simulink model "firmware"  (R2020a)
settings: Solver=FixedStepAuto  StartTime=0.0  StopTime=10.0  FixedStep=1e-3  RelTol=1e-3  EnableMultiTasking=on
undefined symbols (not defined in the file): A0, A1, D0, D1, D10, D11, D12, D13, D2, D3, D4, D5, D6, D7, D8, D9, magnitude, PTA0, PTA1, PTA2, PTB2, PTB23, PTB3, PTB9, PTC16, PTC17, PTC2, PTC3, PTC4, PTD0, PTD1, PTD2, PTD3
libraries: etargetslib x35, frdmk64flib x23, dspstat3 x1
(part 1 of 2)
settings Model: ExtModeTrigDuration=5  Creator=eotte  LastModifiedBy=rafit
settings OptimizationCC: EnhancedBackFolding=on  PassReuseOutputArgsAs=Individual arguments  ZeroExternalMemoryAtStartup=off  ZeroInternalMemoryAtStartup=off  MaxStackSize=64  OptimizeBlockOrder=speed  DifferentSizesBufferReuse=on  OptimizationCustomize=off  EfficientTunableParamExpr=on
settings DebuggingCC: ParameterTunabilityLossMsg=error
settings HardwareCC: ProdBitPerPointer=32  ProdBitPerSizeT=32  ProdBitPerPtrDiffT=32  ProdLargestAtomicInteger=Long  ProdLargestAtomicFloat=Double  ProdWordSize=32  ProdHWDeviceType=ARM Compatible->ARM Cortex
settings SFSimCC: MATLABDynamicMemAlloc=off
settings RTWCC: SystemTargetFile=ert.tlc  HardwareBoard=NXP FRDM-K64F  TemplateMakefile=ert_default_tmf  Toolchain=GNU Tools for ARM Embedded Processors
settings CodeAppCC: ForceParamTrailComments=on  IgnoreCustomStorageClasses=off  OperatorAnnotations=on  SimulinkDataObjDesc=on  SFDataObjDesc=on  InsertBlockDesc=on

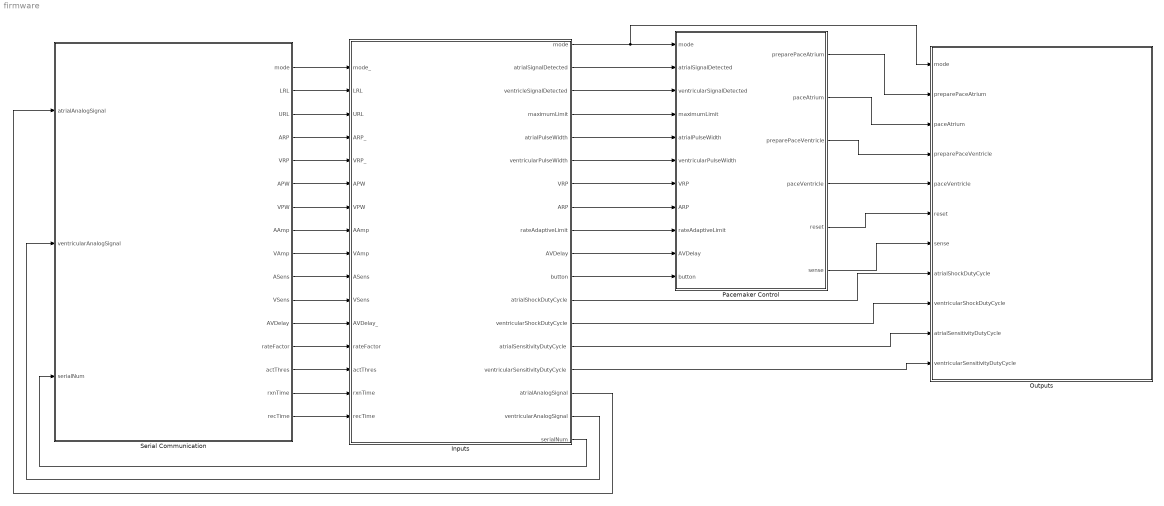
== system firmware ==
  Inputs : Subsystem
  Outputs : Subsystem
  Pacemaker Control : Stateflow chart  TreatAsAtomicUnit=on
  Serial Communication : Subsystem
  wires:
  Pacemaker Control/1(preparePaceAtrium) -> Outputs/2(preparePaceAtrium)
  Pacemaker Control/3(preparePaceVentricle) -> Outputs/4(preparePaceVentricle)
  Pacemaker Control/2(paceAtrium) -> Outputs/3(paceAtrium)
  Pacemaker Control/4(paceVentricle) -> Outputs/5(paceVentricle)
  Inputs/1(mode) -> Pacemaker Control/1(mode), Outputs/1(mode)
  Pacemaker Control/5(reset) -> Outputs/6(reset)
  Inputs/2(atrialSignalDetected) -> Pacemaker Control/2(atrialSignalDetected)
  Inputs/3(ventricleSignalDetected) -> Pacemaker Control/3(ventricularSignalDetected)
  Inputs/15(ventricularSensitivityDutyCycle) -> Outputs/11(ventricularSensitivityDutyCycle)
  Inputs/14(atrialSensitivityDutyCycle) -> Outputs/10(atrialSensitivityDutyCycle)
  Inputs/13(ventricularShockDutyCycle) -> Outputs/9(ventricularShockDutyCycle)
  Inputs/12(atrialShockDutyCycle) -> Outputs/8(atrialShockDutyCycle)
  Inputs/4(maximumLimit) -> Pacemaker Control/4(maximumLimit)
  Inputs/5(atrialPulseWidth) -> Pacemaker Control/5(atrialPulseWidth)
  Inputs/6(ventricularPulseWidth) -> Pacemaker Control/6(ventricularPulseWidth)
  Inputs/7(VRP) -> Pacemaker Control/7(VRP)
  Inputs/8(ARP) -> Pacemaker Control/8(ARP)
  Pacemaker Control/6(sense) -> Outputs/7(sense)
  Serial Communication/1(mode) -> Inputs/1(mode_)
  Serial Communication/2(LRL) -> Inputs/2(LRL)
  Serial Communication/3(URL) -> Inputs/3(URL)
  Serial Communication/4(ARP) -> Inputs/4(ARP_)
  Serial Communication/5(VRP) -> Inputs/5(VRP_)
  Serial Communication/6(APW) -> Inputs/6(APW)
  Serial Communication/7(VPW) -> Inputs/7(VPW)
  Serial Communication/8(AAmp) -> Inputs/8(AAmp)
  Serial Communication/9(VAmp) -> Inputs/9(VAmp)
  Serial Communication/10(ASens) -> Inputs/10(ASens)
  Serial Communication/11(VSens) -> Inputs/11(VSens)
  Inputs/18(serialNum) -> Serial Communication/3(serialNum)
  Inputs/17(ventricularAnalogSignal) -> Serial Communication/2(ventricularAnalogSignal)
  Inputs/16(atrialAnalogSignal) -> Serial Communication/1(atrialAnalogSignal)
  Serial Communication/12(AVDelay) -> Inputs/12(AVDelay_)
  Serial Communication/13(rateFactor) -> Inputs/13(rateFactor)
  Serial Communication/14(actThres) -> Inputs/14(actThres)
  Serial Communication/15(rxnTime) -> Inputs/15(rxnTime)
  Serial Communication/16(recTime) -> Inputs/16(recTime)
  Inputs/9(rateAdaptiveLimit) -> Pacemaker Control/9(rateAdaptiveLimit)
  Inputs/10(AVDelay) -> Pacemaker Control/10(AVDelay)
  Inputs/11(button) -> Pacemaker Control/11(button)

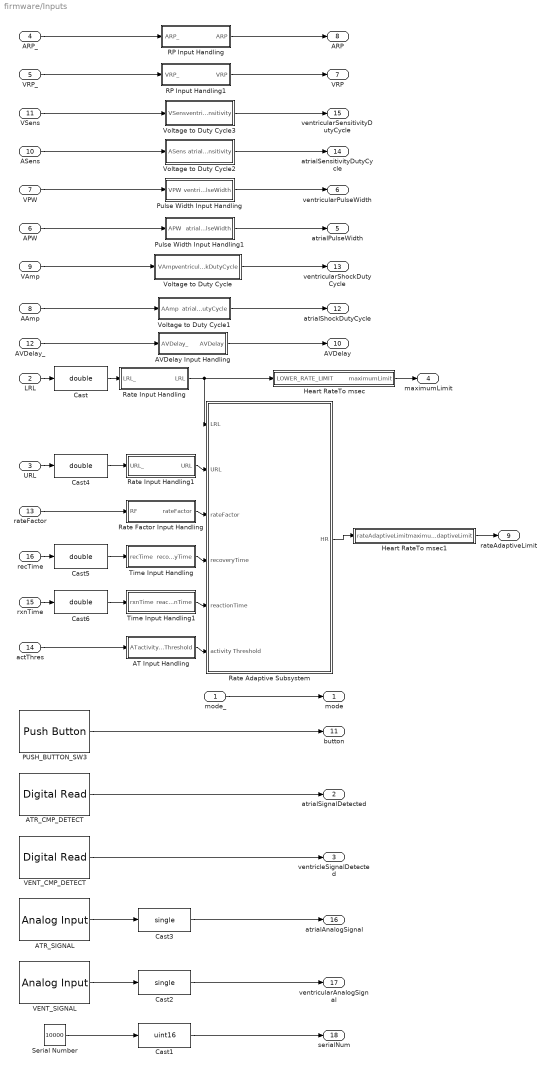
== system firmware/Inputs ==
  mode_ : Inport
  LRL : Inport  Port=2
  URL : Inport  Port=3
  ARP_ : Inport  Port=4
  VRP_ : Inport  Port=5
  APW : Inport  Port=6
  VPW : Inport  Port=7
  AAmp : Inport  Port=8
  VAmp : Inport  Port=9
  ASens : Inport  Port=10
  VSens : Inport  Port=11
  AVDelay_ : Inport  Port=12
  rateFactor : Inport  Port=13
  actThres : Inport  Port=14
  rxnTime : Inport  Port=15
  recTime : Inport  Port=16
  AT Input Handling : Subsystem
  ATR_CMP_DETECT : frdmk64flib/Digital Read  Whichpin=PTC16 (D0)  SampleTime=-1
  ATR_SIGNAL : frdmk64flib/Analog Input  Whichpin=PTB2 (A0)  SampleTime=-1
  AVDelay Input Handling : Subsystem
  Cast{,4..6} (4 alike) : DataTypeConversion  OutDataTypeStr=double  RndMeth=Nearest
  Cast1 : DataTypeConversion  OutDataTypeStr=uint16  RndMeth=Nearest
  Cast2 : DataTypeConversion  OutDataTypeStr=single  RndMeth=Nearest
  Cast3 : DataTypeConversion  OutDataTypeStr=single  RndMeth=Nearest
  Heart RateTo msec : Subsystem
  Heart RateTo msec1 : Subsystem
  PUSH_BUTTON_SW3 : frdmk64flib/Push Button  Whichswitch=SW3  SampleTime1=-1
  Pulse Width Input Handling : Subsystem
  Pulse Width Input Handling1 : Subsystem
  RP Input Handling : Subsystem
  RP Input Handling1 : Subsystem
  Rate Adaptive Subsystem : Subsystem
  Rate Factor Input Handling : Subsystem
  Rate Input Handling : Subsystem
  Rate Input Handling1 : Subsystem
  Serial Number : Constant  Value=10000
  Time Input Handling : Subsystem
  Time Input Handling1 : Subsystem
  VENT_CMP_DETECT : frdmk64flib/Digital Read  Whichpin=PTC17 (D1)  SampleTime=-1
  VENT_SIGNAL : frdmk64flib/Analog Input  Whichpin=PTB3 (A1)  SampleTime=-1
  Voltage to Duty Cycle : Subsystem
  Voltage to Duty Cycle1 : Subsystem
  Voltage to Duty Cycle2 : Subsystem
  Voltage to Duty Cycle3 : Subsystem
  mode : Outport
  atrialSignalDetected : Outport  Port=2
  ventricleSignalDetected : Outport  Port=3
  maximumLimit : Outport  Port=4
  atrialPulseWidth : Outport  Port=5
  ventricularPulseWidth : Outport  Port=6
  VRP : Outport  Port=7
  ARP : Outport  Port=8
  rateAdaptiveLimit : Outport  Port=9
  AVDelay : Outport  Port=10
  button : Outport  Port=11
  atrialShockDutyCycle : Outport  Port=12
  ventricularShockDutyCycle : Outport  Port=13
  atrialSensitivityDutyCycle : Outport  Port=14
  ventricularSensitivityDutyCycle : Outport  Port=15
  atrialAnalogSignal : Outport  Port=16
  ventricularAnalogSignal : Outport  Port=17
  serialNum : Outport  Port=18
  wires:
  mode_/1 -> mode/1
  ATR_CMP_DETECT/1 -> atrialSignalDetected/1
  VENT_CMP_DETECT/1 -> ventricleSignalDetected/1
  AAmp/1 -> Voltage to Duty Cycle1/1(AAmp)
  VAmp/1 -> Voltage to Duty Cycle/1(VAmp)
  VSens/1 -> Voltage to Duty Cycle3/1(VSens)
  ASens/1 -> Voltage to Duty Cycle2/1(ASens)
  VPW/1 -> Pulse Width Input Handling/1(VPW)
  Heart RateTo msec/1(maximumLimit) -> maximumLimit/1
  Voltage to Duty Cycle/1(ventricularShockDutyCycle) -> ventricularShockDutyCycle/1
  Voltage to Duty Cycle1/1(atrialShockDutyCycle) -> atrialShockDutyCycle/1
  Voltage to Duty Cycle3/1(ventricularSensitivity) -> ventricularSensitivityDutyCycle/1
  Voltage to Duty Cycle2/1(atrialSensitivity) -> atrialSensitivityDutyCycle/1
  Pulse Width Input Handling/1(ventricularPulseWidth) -> ventricularPulseWidth/1
  Pulse Width Input Handling1/1(atrialPulseWidth) -> atrialPulseWidth/1
  APW/1 -> Pulse Width Input Handling1/1(APW)
  RP Input Handling1/1(VRP) -> VRP/1
  RP Input Handling/1(ARP) -> ARP/1
  ARP_/1 -> RP Input Handling/1(ARP_)
  VRP_/1 -> RP Input Handling1/1(VRP_)
  Serial Number/1 -> Cast1/1
  ATR_SIGNAL/1 -> Cast3/1
  VENT_SIGNAL/1 -> Cast2/1
  Cast1/1 -> serialNum/1
  Cast2/1 -> ventricularAnalogSignal/1
  Cast3/1 -> atrialAnalogSignal/1
  rateFactor/1 -> Rate Factor Input Handling/1(RF)
  actThres/1 -> AT Input Handling/1(AT)
  Rate Adaptive Subsystem/1(HR) -> Heart RateTo msec1/1(rateAdaptiveLimit)
  Heart RateTo msec1/1(maximumAdaptiveLimit) -> rateAdaptiveLimit/1
  AVDelay_/1 -> AVDelay Input Handling/1(AVDelay_)
  PUSH_BUTTON_SW3/1 -> button/1
  AVDelay Input Handling/1(AVDelay) -> AVDelay/1
  LRL/1 -> Cast/1
  Cast/1 -> Rate Input Handling/1(LRL_)
  Rate Input Handling/1(LRL) -> Heart RateTo msec/1(LOWER_RATE_LIMIT), Rate Adaptive Subsystem/1(LRL)
  Cast4/1 -> Rate Input Handling1/1(URL_)
  Rate Input Handling1/1(URL) -> Rate Adaptive Subsystem/2(URL)
  URL/1 -> Cast4/1
  Rate Factor Input Handling/1(rateFactor) -> Rate Adaptive Subsystem/3(rateFactor)
  Time Input Handling/1(recoveryTime) -> Rate Adaptive Subsystem/4(recoveryTime)
  Time Input Handling1/1(reactionTime) -> Rate Adaptive Subsystem/5(reactionTime)
  AT Input Handling/1(activityThreshold) -> Rate Adaptive Subsystem/6(activity Threshold)
  Cast5/1 -> Time Input Handling/1(recTime)
  recTime/1 -> Cast5/1
  Cast6/1 -> Time Input Handling1/1(rxnTime)
  rxnTime/1 -> Cast6/1

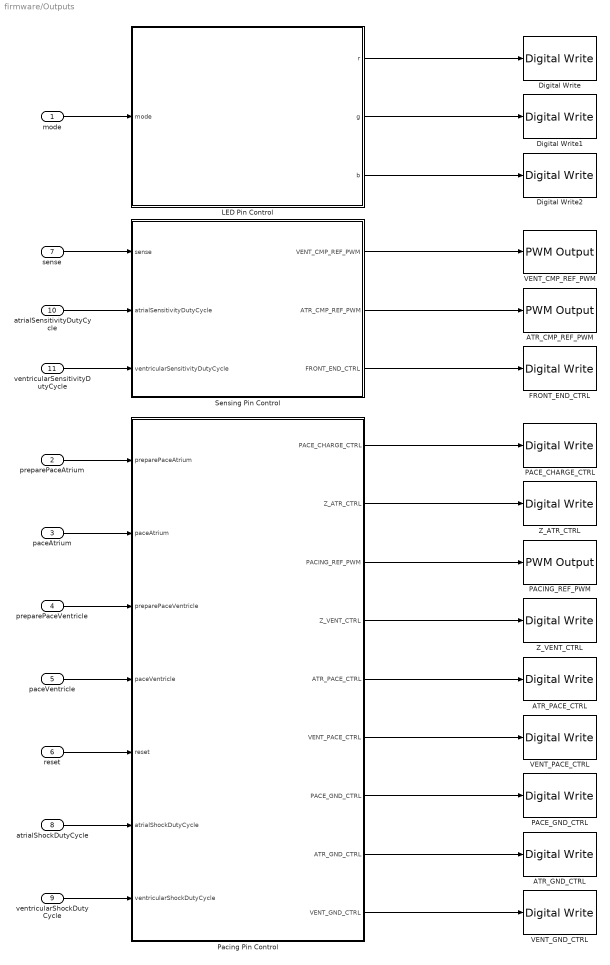
== system firmware/Outputs ==
  mode : Inport
  preparePaceAtrium : Inport  Port=2
  paceAtrium : Inport  Port=3
  preparePaceVentricle : Inport  Port=4
  paceVentricle : Inport  Port=5
  reset : Inport  Port=6
  sense : Inport  Port=7
  atrialShockDutyCycle : Inport  Port=8
  ventricularShockDutyCycle : Inport  Port=9
  atrialSensitivityDutyCycle : Inport  Port=10
  ventricularSensitivityDutyCycle : Inport  Port=11
  ATR_CMP_REF_PWM : frdmk64flib/PWM Output  Whichpin=PTC2 (D6)  InitialFrequency=2000  InitialDutyCycle=0
  ATR_GND_CTRL : frdmk64flib/Digital Write  Whichpin=PTD2 (D11)
  ATR_PACE_CTRL : frdmk64flib/Digital Write  Whichpin=PTA0 (D8)
  Digital Write : frdmk64flib/Digital Write  Whichpin=RED_LED
  Digital Write1 : frdmk64flib/Digital Write  Whichpin=GREEN_LED
  Digital Write2 : frdmk64flib/Digital Write  Whichpin=BLUE_LED
  FRONT_END_CTRL : frdmk64flib/Digital Write  Whichpin=PTD1 (D13)
  LED Pin Control : Stateflow chart  TreatAsAtomicUnit=on
  PACE_CHARGE_CTRL : frdmk64flib/Digital Write  Whichpin=PTB9 (D2)
  PACE_GND_CTRL : frdmk64flib/Digital Write  Whichpin=PTD0 (D10)
  PACING_REF_PWM : frdmk64flib/PWM Output  Whichpin=PTA2 (D5)  InitialFrequency=2000  InitialDutyCycle=0
  Pacing Pin Control : Stateflow chart  TreatAsAtomicUnit=on
      settings: PortSchema="{\"entries\":[{\"content\":{\"sides\":[{\"content\":{\"connectorIds\":[\"In1\",\"In2\",\"In3\",\"In4\",\"In5\",\"In6\",\"In7\"]},\"type\":\"ConnectorPlacement.EquallySpacedRectSide\",\"uuid\":\"92253962-87e9-4e7c-bcdb-24e58fe0c055\"},{\"content\":{\"connectorIds\":[\"Out2\",\"Out8\",\"Out5\",\"Out9\",\"Out3\",\"Out7\",\"Out4\",\"Out1\",\"Out6\"],\"side\":\"RIGHT\"},\"type\":\"ConnectorPlacement.EquallySpacedRectSide\",\"uuid\":\"4cb9541d-32ff-4bb4-8e4b-d9f1d7e76c76\"},{\"content\":{\"connectorIds\":[],\"side\":\"TOP\"},\"type\":\"ConnectorPlacement.EquallySpacedRectSide\",\"uuid\":\"cc690cb9-25b8-4ee8-ae3f-a22909f5e3a8\"},{\"content\":{\"connectorIds\":[],\"side\":\"BOTTOM\"},\"type\":\"ConnectorPlacement.EquallySpacedRectSide\",\"uuid\":\"0aa6c860-c953-4b2e-baf5-040a508b9d07\"}]},\"type\":\"ConnectorPlacement.EquallySpacedConnector\",\"uuid\":\"d7c6b2d5-ade3-439b-b1ea-d68e76d328ac\"}],\"packageUris\":[\"http://schema.mathworks.com/mf0/Connector/19700101\"],\"version\":\"1.0\"}"
  Sensing Pin Control : Stateflow chart  TreatAsAtomicUnit=on
      settings: PortSchema="{\"entries\":[{\"content\":{\"sides\":[{\"content\":{\"connectorIds\":[\"In1\",\"In2\",\"In3\"]},\"type\":\"ConnectorPlacement.EquallySpacedRectSide\",\"uuid\":\"f0f6a072-4109-4fa4-bc82-6d6350130513\"},{\"content\":{\"connectorIds\":[\"Out3\",\"Out2\",\"Out1\"],\"side\":\"RIGHT\"},\"type\":\"ConnectorPlacement.EquallySpacedRectSide\",\"uuid\":\"04a191da-9ef7-404f-bbc7-e2275fa0f798\"},{\"content\":{\"connectorIds\":[],\"side\":\"TOP\"},\"type\":\"ConnectorPlacement.EquallySpacedRectSide\",\"uuid\":\"3258143e-ec04-4818-a8fd-7397dd93120a\"}]},\"type\":\"ConnectorPlacement.EquallySpacedConnector\",\"uuid\":\"abd9187b-7230-471c-b20b-6fa4748c984d\"}],\"packageUris\":[\"http://schema.mathworks.com/mf0/Connector/19700101\"],\"version\":\"1.0\"}"
  VENT_CMP_REF_PWM : frdmk64flib/PWM Output  Whichpin=PTA1 (D3)  InitialFrequency=2000  InitialDutyCycle=0
  VENT_GND_CTRL : frdmk64flib/Digital Write  Whichpin=PTD3 (D12)
  VENT_PACE_CTRL : frdmk64flib/Digital Write  Whichpin=PTC4 (D9)
  Z_ATR_CTRL : frdmk64flib/Digital Write  Whichpin=PTB23 (D4)
  Z_VENT_CTRL : frdmk64flib/Digital Write  Whichpin=PTC3 (D7)
  wires:
  preparePaceAtrium/1 -> Pacing Pin Control/1(preparePaceAtrium)
  paceAtrium/1 -> Pacing Pin Control/2(paceAtrium)
  preparePaceVentricle/1 -> Pacing Pin Control/3(preparePaceVentricle)
  paceVentricle/1 -> Pacing Pin Control/4(paceVentricle)
  Pacing Pin Control/1(ATR_GND_CTRL) -> ATR_GND_CTRL/1
  Pacing Pin Control/2(PACE_CHARGE_CTRL) -> PACE_CHARGE_CTRL/1
  Pacing Pin Control/3(ATR_PACE_CTRL) -> ATR_PACE_CTRL/1
  Pacing Pin Control/5(PACING_REF_PWM) -> PACING_REF_PWM/1
  Pacing Pin Control/8(Z_ATR_CTRL) -> Z_ATR_CTRL/1
  Pacing Pin Control/4(PACE_GND_CTRL) -> PACE_GND_CTRL/1
  Pacing Pin Control/6(VENT_GND_CTRL) -> VENT_GND_CTRL/1
  Pacing Pin Control/9(Z_VENT_CTRL) -> Z_VENT_CTRL/1
  Pacing Pin Control/7(VENT_PACE_CTRL) -> VENT_PACE_CTRL/1
  reset/1 -> Pacing Pin Control/5(reset)
  atrialShockDutyCycle/1 -> Pacing Pin Control/6(atrialShockDutyCycle)
  ventricularShockDutyCycle/1 -> Pacing Pin Control/7(ventricularShockDutyCycle)
  LED Pin Control/2(g) -> Digital Write1/1
  LED Pin Control/1(r) -> Digital Write/1
  LED Pin Control/3(b) -> Digital Write2/1
  mode/1 -> LED Pin Control/1(mode)
  sense/1 -> Sensing Pin Control/1(sense)
  atrialSensitivityDutyCycle/1 -> Sensing Pin Control/2(atrialSensitivityDutyCycle)
  ventricularSensitivityDutyCycle/1 -> Sensing Pin Control/3(ventricularSensitivityDutyCycle)
  Sensing Pin Control/1(FRONT_END_CTRL) -> FRONT_END_CTRL/1
  Sensing Pin Control/2(ATR_CMP_REF_PWM) -> ATR_CMP_REF_PWM/1
  Sensing Pin Control/3(VENT_CMP_REF_PWM) -> VENT_CMP_REF_PWM/1

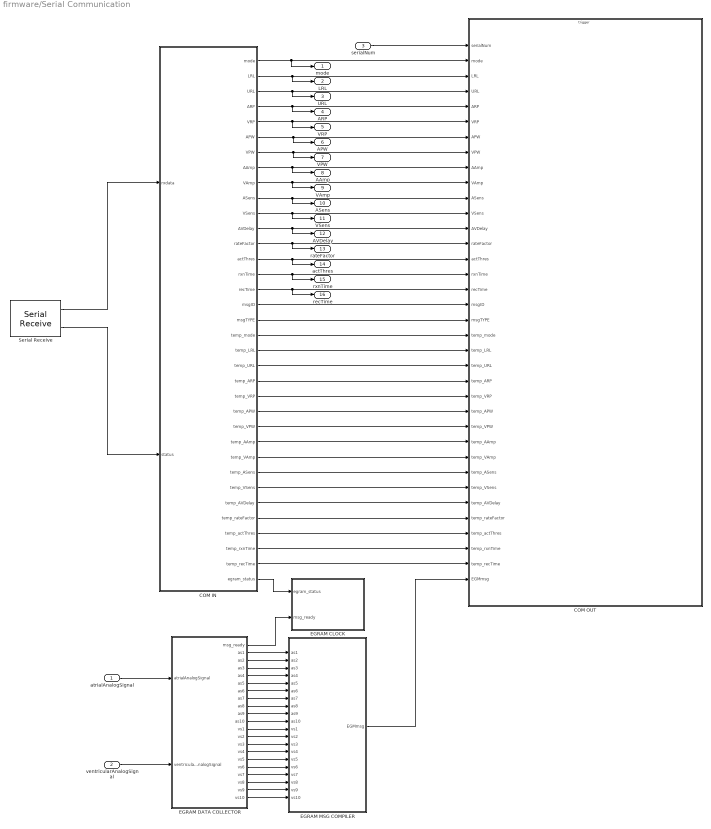
== system firmware/Serial Communication ==
  atrialAnalogSignal : Inport
  ventricularAnalogSignal : Inport  Port=2
  serialNum : Inport  Port=3
  COM IN : Stateflow chart  TreatAsAtomicUnit=on
      settings: PortSchema="{\"entries\":[{\"content\":{\"sides\":[{\"content\":{\"connectorIds\":[\"In1\",\"In2\"]},\"type\":\"ConnectorPlacement.EquallySpacedRectSide\",\"uuid\":\"2e8e9e18-d37c-4b73-b0dd-3e22f2864207\"},{\"content\":{\"connectorIds\":[\"Out1\",\"Out2\",\"Out3\",\"Out4\",\"Out5\",\"Out6\",\"Out7\",\"Out8\",\"Out9\",\"Out10\",\"Out11\",\"Out12\",\"Out13\",\"Out14\",\"Out15\",\"Out16\",\"Out28\",\"Out29\",\"Out17\",\"Out18\",\"Out19\",\"Out20\",\"Out21\",\"Out22\",\"Out23\",\"Out24\",\"Out25\",\"Out26\",\"Out27\",\"Out30\",\"Out31\",\"Out32\",\"Out33\",\"Out34\",\"Out35\"],\"side\":\"RIGHT\"},\"type\":\"ConnectorPlacement.EquallySpacedRectSide\",\"uuid\":\"4c9bee01-a377-43c4-9bd2-1da39583f7b1\"},{\"content\":{\"connectorIds\":[],\"side\":\"TOP\"},\"type\":\"ConnectorPlacement.EquallySpacedRectSide\",\"uuid\":\"f3e8c630-a6ea-4f37-b829-1068b53873bf\"},{\"content\":{\"connectorIds\":[],\"side\":\"BOTTOM\"},\"type\":\"ConnectorPlacement.EquallySpacedRectSide\",\"uuid\":\"e2f98f06-b9c7-4ad9-9fdf-47a7e91a95c4\"}]},\"type\":\"ConnectorPlacement.EquallySpacedConnector\",\"uuid\":\"8e1bc096-629b-4ab2-88c2-6836d8378271\"}],\"packageUris\":[\"http://schema.mathworks.com/mf0/Connector/19700101\"],\"version\":\"1.0\"}"
  COM OUT : Subsystem  TreatAsAtomicUnit=on
  EGRAM CLOCK : Stateflow chart  TreatAsAtomicUnit=on
  EGRAM DATA COLLECTOR : Stateflow chart  TreatAsAtomicUnit=on
      settings: PortSchema="{\"entries\":[{\"content\":{\"sides\":[{\"content\":{\"connectorIds\":[\"In1\",\"In2\"]},\"type\":\"ConnectorPlacement.EquallySpacedRectSide\",\"uuid\":\"97e1670e-7108-4d44-b2cd-721317f0ea01\"},{\"content\":{\"connectorIds\":[\"Out1\",\"Out2\",\"Out3\",\"Out4\",\"Out9\",\"Out10\",\"Out11\",\"Out12\",\"Out13\",\"Out14\",\"Out8\",\"Out5\",\"Out6\",\"Out7\",\"Out16\",\"Out17\",\"Out18\",\"Out19\",\"Out20\",\"Out21\",\"Out15\"],\"side\":\"RIGHT\"},\"type\":\"ConnectorPlacement.EquallySpacedRectSide\",\"uuid\":\"43d6a441-c68e-4a27-91a0-990e1296c4d1\"},{\"content\":{\"connectorIds\":[],\"side\":\"TOP\"},\"type\":\"ConnectorPlacement.EquallySpacedRectSide\",\"uuid\":\"c7be9cee-947c-49b5-a7f8-da78c79fbdaa\"}]},\"type\":\"ConnectorPlacement.EquallySpacedConnector\",\"uuid\":\"a175dd55-c9cb-4f10-b1e9-b74267d4f2a4\"}],\"packageUris\":[\"http://schema.mathworks.com/mf0/Connector/19700101\"],\"version\":\"1.0\"}"
  EGRAM MSG COMPILER : Subsystem
  Serial Receive : frdmk64flib/Serial Receive  SCIModule=0  Baudrate=uint32(9600)  Parity=None  StopBits=1  HardwareFlowControl=None  ByteOrder=LittleEndian  DataType=uint8  DataLength=82  BlockingMode=off  OutputStatus=on  SampleTime=-1
  mode : Outport
  LRL : Outport  Port=2
  URL : Outport  Port=3
  ARP : Outport  Port=4
  VRP : Outport  Port=5
  APW : Outport  Port=6
  VPW : Outport  Port=7
  AAmp : Outport  Port=8
  VAmp : Outport  Port=9
  ASens : Outport  Port=10
  VSens : Outport  Port=11
  AVDelay : Outport  Port=12
  rateFactor : Outport  Port=13
  actThres : Outport  Port=14
  rxnTime : Outport  Port=15
  recTime : Outport  Port=16
  wires:
  Serial Receive/1 -> COM IN/1(rxdata)
  Serial Receive/2 -> COM IN/2(status)
  COM IN/17(temp_mode) -> COM OUT/20(temp_mode)
  COM IN/18(temp_LRL) -> COM OUT/21(temp_LRL)
  COM IN/7(VPW) -> VPW/1, COM OUT/8(VPW)
  COM IN/28(msgID) -> COM OUT/18(msgID)
  COM IN/29(msgTYPE) -> COM OUT/19(msgTYPE)
  COM IN/19(temp_URL) -> COM OUT/22(temp_URL)
  COM IN/20(temp_ARP) -> COM OUT/23(temp_ARP)
  COM IN/21(temp_VRP) -> COM OUT/24(temp_VRP)
  COM IN/22(temp_APW) -> COM OUT/25(temp_APW)
  COM IN/23(temp_VPW) -> COM OUT/26(temp_VPW)
  COM IN/24(temp_AAmp) -> COM OUT/27(temp_AAmp)
  COM IN/25(temp_VAmp) -> COM OUT/28(temp_VAmp)
  COM IN/26(temp_ASens) -> COM OUT/29(temp_ASens)
  COM IN/27(temp_VSens) -> COM OUT/30(temp_VSens)
  serialNum/1 -> COM OUT/1(serialNum)
  atrialAnalogSignal/1 -> EGRAM DATA COLLECTOR/1(atrialAnalogSignal)
  ventricularAnalogSignal/1 -> EGRAM DATA COLLECTOR/2(ventricularAnalogSignal)
  EGRAM DATA COLLECTOR/1(msg_ready) -> EGRAM CLOCK/2(msg_ready)
  EGRAM MSG COMPILER/1(EGMmsg) -> COM OUT/36(EGMmsg)
  EGRAM DATA COLLECTOR/2(as1) -> EGRAM MSG COMPILER/1(as1)
  EGRAM DATA COLLECTOR/3(as2) -> EGRAM MSG COMPILER/2(as2)
  EGRAM DATA COLLECTOR/4(as3) -> EGRAM MSG COMPILER/3(as3)
  EGRAM DATA COLLECTOR/5(vs1) -> EGRAM MSG COMPILER/11(vs1)
  EGRAM DATA COLLECTOR/6(vs2) -> EGRAM MSG COMPILER/12(vs2)
  EGRAM DATA COLLECTOR/7(vs3) -> EGRAM MSG COMPILER/13(vs3)
  COM IN/35(egram_status) -> EGRAM CLOCK/1(egram_status)
  EGRAM DATA COLLECTOR/9(as4) -> EGRAM MSG COMPILER/4(as4)
  EGRAM DATA COLLECTOR/10(as5) -> EGRAM MSG COMPILER/5(as5)
  EGRAM DATA COLLECTOR/11(as6) -> EGRAM MSG COMPILER/6(as6)
  EGRAM DATA COLLECTOR/12(as7) -> EGRAM MSG COMPILER/7(as7)
  EGRAM DATA COLLECTOR/13(as8) -> EGRAM MSG COMPILER/8(as8)
  EGRAM DATA COLLECTOR/14(as9) -> EGRAM MSG COMPILER/9(as9)
  EGRAM DATA COLLECTOR/8(as10) -> EGRAM MSG COMPILER/10(as10)
  EGRAM DATA COLLECTOR/16(vs4) -> EGRAM MSG COMPILER/14(vs4)
  EGRAM DATA COLLECTOR/17(vs5) -> EGRAM MSG COMPILER/15(vs5)
  EGRAM DATA COLLECTOR/18(vs6) -> EGRAM MSG COMPILER/16(vs6)
  EGRAM DATA COLLECTOR/19(vs7) -> EGRAM MSG COMPILER/17(vs7)
  EGRAM DATA COLLECTOR/20(vs8) -> EGRAM MSG COMPILER/18(vs8)
  EGRAM DATA COLLECTOR/21(vs9) -> EGRAM MSG COMPILER/19(vs9)
  EGRAM DATA COLLECTOR/15(vs10) -> EGRAM MSG COMPILER/20(vs10)
  COM IN/1(mode) -> mode/1, COM OUT/2(mode)
  COM IN/2(LRL) -> LRL/1, COM OUT/3(LRL)
  COM IN/3(URL) -> URL/1, COM OUT/4(URL)
  COM IN/4(ARP) -> ARP/1, COM OUT/5(ARP)
  COM IN/5(VRP) -> VRP/1, COM OUT/6(VRP)
  COM IN/6(APW) -> APW/1, COM OUT/7(APW)
  COM IN/8(AAmp) -> AAmp/1, COM OUT/9(AAmp)
  COM IN/9(VAmp) -> VAmp/1, COM OUT/10(VAmp)
  COM IN/10(ASens) -> COM OUT/11(ASens), ASens/1
  COM IN/11(VSens) -> VSens/1, COM OUT/12(VSens)
  COM IN/12(AVDelay) -> AVDelay/1, COM OUT/13(AVDelay)
  COM IN/13(rateFactor) -> rateFactor/1, COM OUT/14(rateFactor)
  COM IN/14(actThres) -> actThres/1, COM OUT/15(actThres)
  COM IN/15(rxnTime) -> rxnTime/1, COM OUT/16(rxnTime)
  COM IN/16(recTime) -> recTime/1, COM OUT/17(recTime)
  COM IN/30(temp_AVDelay) -> COM OUT/31(temp_AVDelay)
  COM IN/31(temp_rateFactor) -> COM OUT/32(temp_rateFactor)
  COM IN/32(temp_actThres) -> COM OUT/33(temp_actThres)
  COM IN/33(temp_rxnTime) -> COM OUT/34(temp_rxnTime)
  COM IN/34(temp_recTime) -> COM OUT/35(temp_recTime)

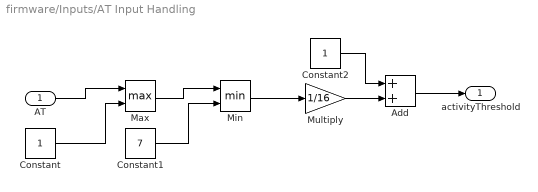
== system firmware/Inputs/AT Input Handling ==
  AT : Inport
  Add : Sum
  Constant : Constant
  Constant1 : Constant  Value=7
  Constant2 : Constant
  Max : MinMax  Function=max  Inputs=2
  Min : MinMax  Inputs=2
  Multiply : Gain  Gain=1/16
  activityThreshold : Outport
  wires:
  Max/1 -> Min/1
  AT/1 -> Max/1
  Min/1 -> Multiply/1
  Constant/1 -> Max/2
  Constant1/1 -> Min/2
  Constant2/1 -> Add/1
  Multiply/1 -> Add/2
  Add/1 -> activityThreshold/1

== system firmware/Inputs/AVDelay Input Handling ==
  AVDelay_ : Inport
  Constant : Constant  Value=30
  Constant1 : Constant  Value=300
  Max : MinMax  Function=max  Inputs=2
  Min : MinMax  Inputs=2
  AVDelay : Outport
  wires:
  Max/1 -> Min/1
  AVDelay_/1 -> Max/1
  Min/1 -> AVDelay/1
  Constant/1 -> Max/2
  Constant1/1 -> Min/2

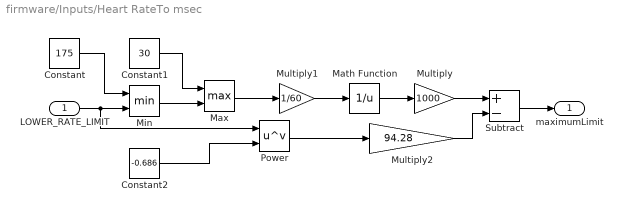
== system firmware/Inputs/Heart RateTo msec ==
  LOWER_RATE_LIMIT : Inport
  Constant : Constant  Value=175
  Constant1 : Constant  Value=30
  Constant2 : Constant  Value=-0.686
  Math Function : Math  Operator=reciprocal  SaturateOnIntegerOverflow=on
  Max : MinMax  Function=max  Inputs=2
  Min : MinMax  Inputs=2
  Multiply : Gain  Gain=1000
  Multiply1 : Gain  Gain=1/60
  Multiply2 : Gain  Gain=94.28
  Power : Math  Operator=pow  OutputSignalType=real  SaturateOnIntegerOverflow=on
  Subtract : Sum  Inputs=+-
  maximumLimit : Outport
  wires:
  Multiply1/1 -> Math Function/1
  Multiply/1 -> Subtract/1
  LOWER_RATE_LIMIT/1 -> Power/1, Min/2
  Min/1 -> Max/2
  Max/1 -> Multiply1/1
  Constant/1 -> Min/1
  Constant1/1 -> Max/1
  Math Function/1 -> Multiply/1
  Subtract/1 -> maximumLimit/1
  Multiply2/1 -> Subtract/2
  Constant2/1 -> Power/2
  Power/1 -> Multiply2/1

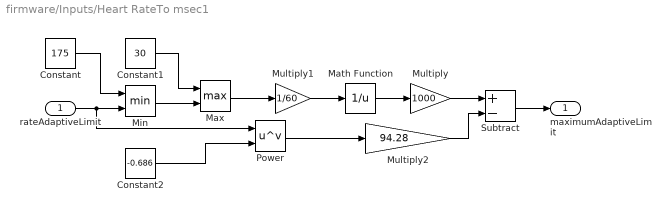
== system firmware/Inputs/Heart RateTo msec1 ==
  rateAdaptiveLimit : Inport
  Constant : Constant  Value=175
  Constant1 : Constant  Value=30
  Constant2 : Constant  Value=-0.686
  Math Function : Math  Operator=reciprocal  SaturateOnIntegerOverflow=on
  Max : MinMax  Function=max  Inputs=2
  Min : MinMax  Inputs=2
  Multiply : Gain  Gain=1000
  Multiply1 : Gain  Gain=1/60
  Multiply2 : Gain  Gain=94.28
  Power : Math  Operator=pow  OutputSignalType=real  SaturateOnIntegerOverflow=on
  Subtract : Sum  Inputs=+-
  maximumAdaptiveLimit : Outport
  wires:
  Multiply1/1 -> Math Function/1
  Multiply/1 -> Subtract/1
  rateAdaptiveLimit/1 -> Power/1, Min/2
  Min/1 -> Max/2
  Max/1 -> Multiply1/1
  Constant/1 -> Min/1
  Constant1/1 -> Max/1
  Math Function/1 -> Multiply/1
  Subtract/1 -> maximumAdaptiveLimit/1
  Multiply2/1 -> Subtract/2
  Constant2/1 -> Power/2
  Power/1 -> Multiply2/1

== system firmware/Inputs/Pulse Width Input Handling ==
  VPW : Inport
  Constant : Constant
  Constant1 : Constant  Value=30
  Max : MinMax  Function=max  Inputs=2
  Min : MinMax  Inputs=2
  ventricularPulseWidth : Outport
  wires:
  Max/1 -> Min/1
  VPW/1 -> Max/1
  Min/1 -> ventricularPulseWidth/1
  Constant/1 -> Max/2
  Constant1/1 -> Min/2

== system firmware/Inputs/Pulse Width Input Handling1 ==
  APW : Inport
  Constant : Constant
  Constant1 : Constant  Value=30
  Max : MinMax  Function=max  Inputs=2
  Min : MinMax  Inputs=2
  atrialPulseWidth : Outport
  wires:
  Max/1 -> Min/1
  APW/1 -> Max/1
  Min/1 -> atrialPulseWidth/1
  Constant/1 -> Max/2
  Constant1/1 -> Min/2

== system firmware/Inputs/RP Input Handling ==
  ARP_ : Inport
  Constant : Constant  Value=150
  Constant1 : Constant  Value=500
  Max : MinMax  Function=max  Inputs=2
  Min : MinMax  Inputs=2
  ARP : Outport
  wires:
  Max/1 -> Min/1
  ARP_/1 -> Max/1
  Min/1 -> ARP/1
  Constant/1 -> Max/2
  Constant1/1 -> Min/2

== system firmware/Inputs/RP Input Handling1 ==
  VRP_ : Inport
  Constant : Constant  Value=150
  Constant1 : Constant  Value=500
  Max : MinMax  Function=max  Inputs=2
  Min : MinMax  Inputs=2
  VRP : Outport
  wires:
  Max/1 -> Min/1
  VRP_/1 -> Max/1
  Min/1 -> VRP/1
  Constant/1 -> Max/2
  Constant1/1 -> Min/2

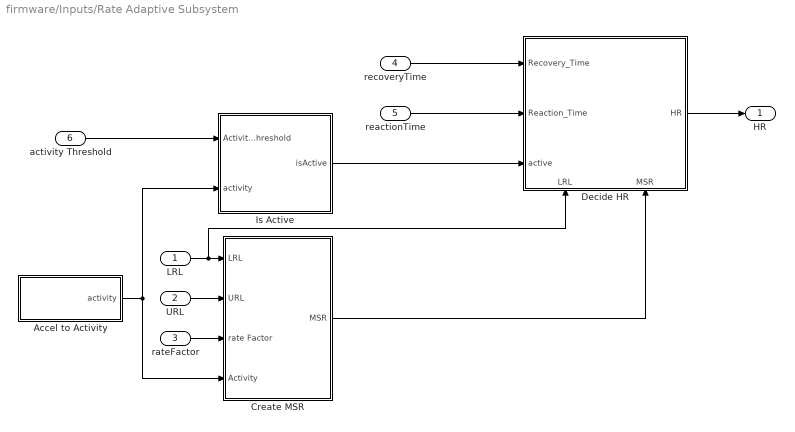
== system firmware/Inputs/Rate Adaptive Subsystem ==
  LRL : Inport
  URL : Inport  Port=2
  rateFactor : Inport  Port=3
  recoveryTime : Inport  Port=4
  reactionTime : Inport  Port=5
  activity Threshold : Inport  Port=6
  Accel to Activity : Subsystem
  Create MSR : Subsystem
  Decide HR : Stateflow chart  TreatAsAtomicUnit=on
      settings: PortSchema="{\"entries\":[{\"content\":{\"sides\":[{\"content\":{\"connectorIds\":[\"In1\",\"In2\",\"In3\"]},\"type\":\"ConnectorPlacement.EquallySpacedRectSide\",\"uuid\":\"9f5eeb57-f726-4755-8de2-368eec17f0e4\"},{\"content\":{\"connectorIds\":[\"Out1\"],\"side\":\"RIGHT\"},\"type\":\"ConnectorPlacement.EquallySpacedRectSide\",\"uuid\":\"be2ce5c8-3baf-46e9-a138-20c0151c1594\"},{\"content\":{\"connectorIds\":[],\"side\":\"TOP\"},\"type\":\"ConnectorPlacement.EquallySpacedRectSide\",\"uuid\":\"e46b4a2e-d259-4de7-b3e3-8621bb25c624\"},{\"content\":{\"connectorIds\":[\"In5\",\"In4\"],\"side\":\"BOTTOM\"},\"type\":\"ConnectorPlacement.EquallySpacedRectSide\",\"uuid\":\"3fec9188-4635-41ac-be97-bcb7e679d5c6\"}]},\"type\":\"ConnectorPlacement.EquallySpacedConnector\",\"uuid\":\"cda5442f-28c8-415b-9799-55bbac838de1\"}],\"packageUris\":[\"http://schema.mathworks.com/mf0/Connector/19700101\"],\"version\":\"1.0\"}"
  Is Active : Stateflow chart  TreatAsAtomicUnit=on
  HR : Outport
  wires:
  Accel to Activity/1(activity) -> Is Active/2(activity), Create MSR/4(Activity)
  rateFactor/1 -> Create MSR/3(rate Factor)
  URL/1 -> Create MSR/2(URL)
  Is Active/1(isActive) -> Decide HR/3(active)
  Create MSR/1(MSR) -> Decide HR/4(MSR)
  Decide HR/1(HR) -> HR/1
  LRL/1 -> Decide HR/5(LRL), Create MSR/1(LRL)
  reactionTime/1 -> Decide HR/2(Reaction_Time)
  recoveryTime/1 -> Decide HR/1(Recovery_Time)
  activity Threshold/1 -> Is Active/1(Activity_Threshold)

== system firmware/Inputs/Rate Factor Input Handling ==
  RF : Inport
  Constant : Constant
  Constant1 : Constant  Value=16
  Max : MinMax  Function=max  Inputs=2
  Min : MinMax  Inputs=2
  rateFactor : Outport
  wires:
  Max/1 -> Min/1
  RF/1 -> Max/1
  Min/1 -> rateFactor/1
  Constant/1 -> Max/2
  Constant1/1 -> Min/2

== system firmware/Inputs/Rate Input Handling ==
  LRL_ : Inport
  Constant : Constant  Value=30
  Constant1 : Constant  Value=175
  Max : MinMax  Function=max  Inputs=2
  Min : MinMax  Inputs=2
  LRL : Outport
  wires:
  Max/1 -> Min/1
  LRL_/1 -> Max/1
  Min/1 -> LRL/1
  Constant/1 -> Max/2
  Constant1/1 -> Min/2

== system firmware/Inputs/Rate Input Handling1 ==
  URL_ : Inport
  Constant : Constant  Value=50
  Constant1 : Constant  Value=175
  Max : MinMax  Function=max  Inputs=2
  Min : MinMax  Inputs=2
  URL : Outport
  wires:
  Max/1 -> Min/1
  URL_/1 -> Max/1
  Min/1 -> URL/1
  Constant/1 -> Max/2
  Constant1/1 -> Min/2

== system firmware/Inputs/Time Input Handling ==
  recTime : Inport
  Constant : Constant
  Constant1 : Constant  Value=240
  Max : MinMax  Function=max  Inputs=2
  Min : MinMax  Inputs=2
  recoveryTime : Outport
  wires:
  Max/1 -> Min/1
  recTime/1 -> Max/1
  Min/1 -> recoveryTime/1
  Constant/1 -> Max/2
  Constant1/1 -> Min/2

== system firmware/Inputs/Time Input Handling1 ==
  rxnTime : Inport
  Constant : Constant
  Constant1 : Constant  Value=50
  Max : MinMax  Function=max  Inputs=2
  Min : MinMax  Inputs=2
  reactionTime : Outport
  wires:
  Max/1 -> Min/1
  rxnTime/1 -> Max/1
  Min/1 -> reactionTime/1
  Constant/1 -> Max/2
  Constant1/1 -> Min/2

== system firmware/Inputs/Voltage to Duty Cycle ==
  VAmp : Inport
  Constant : Constant  Value=0
  Constant1 : Constant  Value=100
  Max : MinMax  Function=max  Inputs=2
  Min : MinMax  Inputs=2
  Multiply : Gain  Gain=100
  Multiply1 : Gain  Gain=0.2
  Round : Rounding  Operator=round
  ventricularShockDutyCycle : Outport
  wires:
  VAmp/1 -> Multiply1/1
  Multiply1/1 -> Multiply/1
  Multiply/1 -> Round/1
  Round/1 -> Max/1
  Max/1 -> Min/1
  Min/1 -> ventricularShockDutyCycle/1
  Constant/1 -> Max/2
  Constant1/1 -> Min/2

== system firmware/Inputs/Voltage to Duty Cycle1 ==
  AAmp : Inport
  Constant : Constant  Value=0
  Constant1 : Constant  Value=100
  Max : MinMax  Function=max  Inputs=2
  Min : MinMax  Inputs=2
  Multiply : Gain  Gain=100
  Multiply1 : Gain  Gain=0.2
  Round : Rounding  Operator=round
  atrialShockDutyCycle : Outport
  wires:
  AAmp/1 -> Multiply1/1
  Multiply1/1 -> Multiply/1
  Multiply/1 -> Round/1
  Round/1 -> Max/1
  Max/1 -> Min/1
  Min/1 -> atrialShockDutyCycle/1
  Constant/1 -> Max/2
  Constant1/1 -> Min/2

== system firmware/Inputs/Voltage to Duty Cycle2 ==
  ASens : Inport
  Constant : Constant  Value=0
  Constant1 : Constant  Value=100
  Max : MinMax  Function=max  Inputs=2
  Min : MinMax  Inputs=2
  Multiply : Gain  Gain=100
  Multiply1 : Gain  Gain=0.2
  Round : Rounding  Operator=round
  atrialSensitivity : Outport
  wires:
  ASens/1 -> Multiply1/1
  Multiply1/1 -> Multiply/1
  Multiply/1 -> Round/1
  Round/1 -> Max/1
  Max/1 -> Min/1
  Min/1 -> atrialSensitivity/1
  Constant/1 -> Max/2
  Constant1/1 -> Min/2

== system firmware/Inputs/Voltage to Duty Cycle3 ==
  VSens : Inport
  Constant : Constant  Value=0
  Constant1 : Constant  Value=100
  Max : MinMax  Function=max  Inputs=2
  Min : MinMax  Inputs=2
  Multiply : Gain  Gain=100
  Multiply1 : Gain  Gain=0.2
  Round : Rounding  Operator=round
  ventricularSensitivity : Outport
  wires:
  VSens/1 -> Multiply1/1
  Multiply1/1 -> Multiply/1
  Multiply/1 -> Round/1
  Round/1 -> Max/1
  Max/1 -> Min/1
  Min/1 -> ventricularSensitivity/1
  Constant/1 -> Max/2
  Constant1/1 -> Min/2

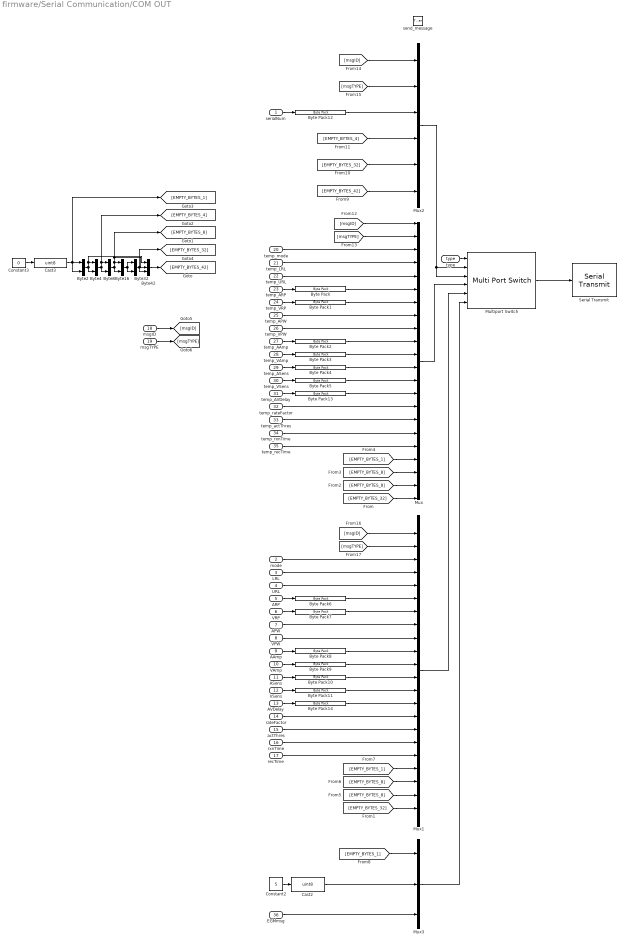
== system firmware/Serial Communication/COM OUT ==
  serialNum : Inport
  mode : Inport  Port=2
  LRL : Inport  Port=3
  URL : Inport  Port=4
  ARP : Inport  Port=5
  VRP : Inport  Port=6
  APW : Inport  Port=7
  VPW : Inport  Port=8
  AAmp : Inport  Port=9
  VAmp : Inport  Port=10
  ASens : Inport  Port=11
  VSens : Inport  Port=12
  AVDelay : Inport  Port=13
  rateFactor : Inport  Port=14
  actThres : Inport  Port=15
  rxnTime : Inport  Port=16
  recTime : Inport  Port=17
  msgID : Inport  Port=18
  msgTYPE : Inport  Port=19
  temp_mode : Inport  Port=20
  temp_LRL : Inport  Port=21
  temp_URL : Inport  Port=22
  temp_ARP : Inport  Port=23
  temp_VRP : Inport  Port=24
  temp_APW : Inport  Port=25
  temp_VPW : Inport  Port=26
  temp_AAmp : Inport  Port=27
  temp_VAmp : Inport  Port=28
  temp_ASens : Inport  Port=29
  temp_VSens : Inport  Port=30
  temp_AVDelay : Inport  Port=31
  temp_rateFactor : Inport  Port=32
  temp_actThres : Inport  Port=33
  temp_rxnTime : Inport  Port=34
  temp_recTime : Inport  Port=35
  EGMmsg : Inport  Port=36
  send_message : TriggerPort  TriggerType=function-call  IsSimulinkFunction=on  FunctionName=send_message  VariantControl=Variant
  Byte Pack{,1,6..7,12..14} (7 alike) : etargetslib/Byte Pack  datatypes={'uint16'}  byteAlign=1
  Byte Pack{2..5,8..11} (8 alike) : etargetslib/Byte Pack  datatypes={'single'}  byteAlign=1
  Byte{2,4,8,16,32} (5 alike) : Mux  Inputs=2
  Byte42 : Mux  Inputs=3
  Cast2 : DataTypeConversion  OutDataTypeStr=uint8  RndMeth=Nearest
  Cast3 : DataTypeConversion  OutDataTypeStr=uint8  RndMeth=Nearest
  Constant2 : Constant  Value=5
  Constant3 : Constant  Value=0
  Multiport Switch : MultiPortSwitch  DataPortOrder=Specify indices  DataPortIndices={1,2,3,4,5}  DiagnosticForDefault=None
  Mux : Mux  Inputs=22
  Mux1 : Mux  Inputs=22
  Mux2 : Mux  Inputs=6
  Mux3 : Mux  Inputs=3
  Serial Transmit : frdmk64flib/Serial Transmit  SCIModule=0  Baudrate=uint32(9600)  Parity=None  StopBits=1  HardwareFlowControl=None  ByteOrder=LittleEndian  BlockingMode=on  OutputStatus=off
  type : ArgIn  ArgumentName=type
  wires:
  temp_mode/1 -> Mux/3
  temp_LRL/1 -> Mux/4
  temp_URL/1 -> Mux/5
  temp_ARP/1 -> Byte Pack/1
  temp_VRP/1 -> Byte Pack1/1
  temp_AAmp/1 -> Byte Pack2/1
  temp_VAmp/1 -> Byte Pack3/1
  temp_ASens/1 -> Byte Pack4/1
  temp_VSens/1 -> Byte Pack5/1
  Mux/1 -> Multiport Switch/4
  Byte Pack5/1 -> Mux/13
  Byte Pack/1 -> Mux/6
  Byte Pack1/1 -> Mux/7
  temp_APW/1 -> Mux/8
  temp_VPW/1 -> Mux/9
  Byte Pack2/1 -> Mux/10
  Byte Pack3/1 -> Mux/11
  Byte Pack4/1 -> Mux/12
  mode/1 -> Mux1/3
  LRL/1 -> Mux1/4
  URL/1 -> Mux1/5
  ARP/1 -> Byte Pack6/1
  VRP/1 -> Byte Pack7/1
  APW/1 -> Mux1/8
  VPW/1 -> Mux1/9
  AAmp/1 -> Byte Pack8/1
  VAmp/1 -> Byte Pack9/1
  ASens/1 -> Byte Pack10/1
  VSens/1 -> Byte Pack11/1
  Mux1/1 -> Multiport Switch/5
  Byte Pack6/1 -> Mux1/6
  Byte Pack7/1 -> Mux1/7
  Byte Pack8/1 -> Mux1/10
  Byte Pack9/1 -> Mux1/11
  Byte Pack10/1 -> Mux1/12
  Byte Pack11/1 -> Mux1/13
  Multiport Switch/1 -> Serial Transmit/1
  serialNum/1 -> Byte Pack12/1
  Byte Pack12/1 -> Mux2/3
  Mux2/1 -> Multiport Switch/3, Multiport Switch/2
  type/1 -> Multiport Switch/1
  Mux3/1 -> Multiport Switch/6
  [EMPTY_BYTES_1] -> Mux3/1
  EGMmsg/1 -> Mux3/3
  Constant2/1 -> Cast2/1
  Cast2/1 -> Mux3/2
  Constant3/1 -> Cast3/1
  Cast3/1 -> Byte2/2, [EMPTY_BYTES_1], Byte2/1
  Byte2/1 -> Byte4/2, Byte42/1, Byte4/1
  Byte4/1 -> Byte8/2, [EMPTY_BYTES_4], Byte8/1
  Byte8/1 -> Byte16/2, [EMPTY_BYTES_8], Byte42/2, Byte16/1
  Byte16/1 -> Byte32/2, Byte32/1
  Byte32/1 -> Byte42/3, [EMPTY_BYTES_32]
  Byte42/1 -> [EMPTY_BYTES_42]
  [EMPTY_BYTES_32] -> Mux/22
  [EMPTY_BYTES_8] -> Mux/21
  [EMPTY_BYTES_8] -> Mux/20
  [EMPTY_BYTES_1] -> Mux/19
  [EMPTY_BYTES_42] -> Mux2/6
  [EMPTY_BYTES_32] -> Mux2/5
  [EMPTY_BYTES_4] -> Mux2/4
  msgID/1 -> [msgID]
  msgTYPE/1 -> [msgTYPE]
  [msgID] -> Mux/1
  [msgTYPE] -> Mux/2
  [msgID] -> Mux2/1
  [msgTYPE] -> Mux2/2
  [msgID] -> Mux1/1
  [msgTYPE] -> Mux1/2
  temp_rateFactor/1 -> Mux/15
  temp_actThres/1 -> Mux/16
  temp_rxnTime/1 -> Mux/17
  temp_recTime/1 -> Mux/18
  Byte Pack13/1 -> Mux/14
  temp_AVDelay/1 -> Byte Pack13/1
  [EMPTY_BYTES_8] -> Mux1/21
  [EMPTY_BYTES_8] -> Mux1/20
  [EMPTY_BYTES_1] -> Mux1/19
  [EMPTY_BYTES_32] -> Mux1/22
  Byte Pack14/1 -> Mux1/14
  AVDelay/1 -> Byte Pack14/1
  rateFactor/1 -> Mux1/15
  actThres/1 -> Mux1/16
  rxnTime/1 -> Mux1/17
  recTime/1 -> Mux1/18

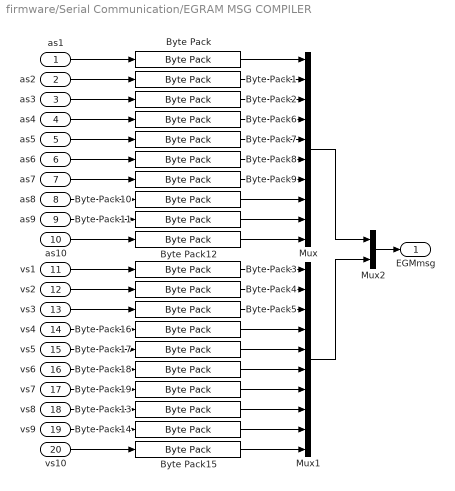
== system firmware/Serial Communication/EGRAM MSG COMPILER ==
  as1 : Inport
  as2 : Inport  Port=2
  as3 : Inport  Port=3
  as4 : Inport  Port=4
  as5 : Inport  Port=5
  as6 : Inport  Port=6
  as7 : Inport  Port=7
  as8 : Inport  Port=8
  as9 : Inport  Port=9
  as10 : Inport  Port=10
  vs1 : Inport  Port=11
  vs2 : Inport  Port=12
  vs3 : Inport  Port=13
  vs4 : Inport  Port=14
  vs5 : Inport  Port=15
  vs6 : Inport  Port=16
  vs7 : Inport  Port=17
  vs8 : Inport  Port=18
  vs9 : Inport  Port=19
  vs10 : Inport  Port=20
  Byte Pack{,1..19} (20 alike) : etargetslib/Byte Pack  datatypes={'single'}  byteAlign=1
  Mux : Mux  Inputs=10
  Mux1 : Mux  Inputs=10
  Mux2 : Mux  Inputs=2
  EGMmsg : Outport
  wires:
  Mux/1 -> Mux2/1
  Byte Pack1/1 -> Mux/2
  Byte Pack/1 -> Mux/1
  as1/1 -> Byte Pack/1
  Byte Pack2/1 -> Mux/3
  as3/1 -> Byte Pack2/1
  as2/1 -> Byte Pack1/1
  vs3/1 -> Byte Pack5/1
  vs2/1 -> Byte Pack4/1
  vs1/1 -> Byte Pack3/1
  Mux1/1 -> Mux2/2
  Mux2/1 -> EGMmsg/1
  Byte Pack3/1 -> Mux1/1
  Byte Pack4/1 -> Mux1/2
  Byte Pack5/1 -> Mux1/3
  Byte Pack16/1 -> Mux1/4
  Byte Pack17/1 -> Mux1/5
  Byte Pack18/1 -> Mux1/6
  Byte Pack19/1 -> Mux1/7
  Byte Pack13/1 -> Mux1/8
  Byte Pack14/1 -> Mux1/9
  Byte Pack15/1 -> Mux1/10
  Byte Pack6/1 -> Mux/4
  Byte Pack7/1 -> Mux/5
  Byte Pack8/1 -> Mux/6
  Byte Pack9/1 -> Mux/7
  Byte Pack10/1 -> Mux/8
  Byte Pack11/1 -> Mux/9
  Byte Pack12/1 -> Mux/10
  as10/1 -> Byte Pack12/1
  as9/1 -> Byte Pack11/1
  as8/1 -> Byte Pack10/1
  as7/1 -> Byte Pack9/1
  as6/1 -> Byte Pack8/1
  as5/1 -> Byte Pack7/1
  as4/1 -> Byte Pack6/1
  vs4/1 -> Byte Pack16/1
  vs5/1 -> Byte Pack17/1
  vs6/1 -> Byte Pack18/1
  vs7/1 -> Byte Pack19/1
  vs8/1 -> Byte Pack13/1
  vs9/1 -> Byte Pack14/1
  vs10/1 -> Byte Pack15/1

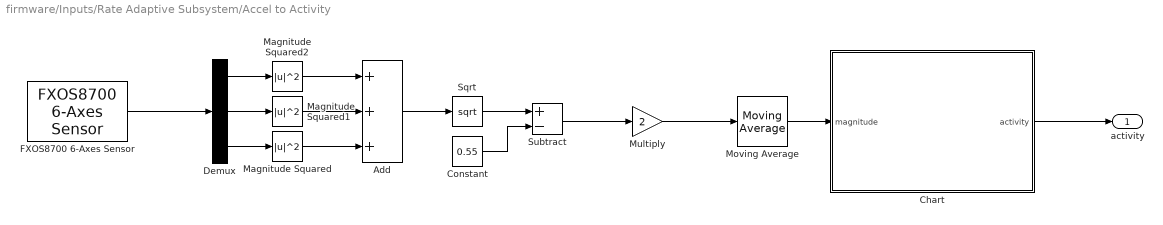
== system firmware/Inputs/Rate Adaptive Subsystem/Accel to Activity ==
  Add : Sum  Inputs=+++
  Chart : Stateflow chart  TreatAsAtomicUnit=on
  Constant : Constant  Value=0.55
  Demux : Demux  Outputs=3
  FXOS8700 6-Axes Sensor : frdmk64flib/FXOS8700 6-Axes Sensor  Activesensor=Accelerometer only  ODR=100Hz  HybridODR=400Hz  Accelfullrange=-4g to +4g  SampleTime=0.002
  Magnitude Squared : Math  Operator=magnitude^2  SaturateOnIntegerOverflow=on
  Magnitude Squared1 : Math  Operator=magnitude^2  SaturateOnIntegerOverflow=on
  Magnitude Squared2 : Math  Operator=magnitude^2  SaturateOnIntegerOverflow=on
  Moving Average : dspstat3/Moving Average  Method=Sliding window  ForgettingFactorPort=off  SpecifyWindowLength=on  WindowLength=1000  ForgettingFactor=0.9  SimulateUsing=Code generation
  Multiply : Gain  Gain=2
  Sqrt : Sqrt  SaturateOnIntegerOverflow=on
  Subtract : Sum  Inputs=+-
  activity : Outport
  wires:
  Demux/3 -> Magnitude Squared/1
  Demux/1 -> Magnitude Squared2/1
  Magnitude Squared1/1 -> Add/2
  Magnitude Squared2/1 -> Add/1
  Magnitude Squared/1 -> Add/3
  Demux/2 -> Magnitude Squared1/1
  FXOS8700 6-Axes Sensor/1 -> Demux/1
  Add/1 -> Sqrt/1
  Sqrt/1 -> Subtract/1
  Multiply/1 -> Moving Average/1
  Subtract/1 -> Multiply/1
  Chart/1(activity) -> activity/1
  Moving Average/1 -> Chart/1(magnitude)
  Constant/1 -> Subtract/2

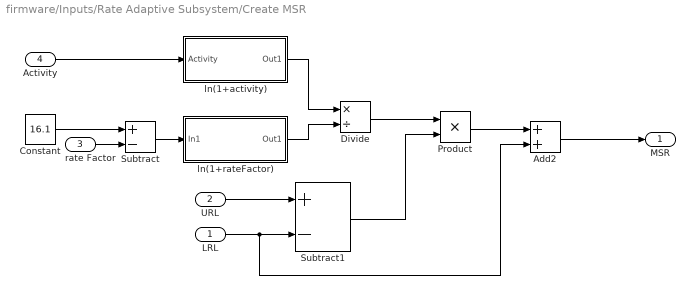
== system firmware/Inputs/Rate Adaptive Subsystem/Create MSR ==
  LRL : Inport
  URL : Inport  Port=2
  rate Factor : Inport  Port=3
  Activity : Inport  Port=4
  Add2 : Sum
  Constant : Constant  Value=16.1
  Divide : Product  Inputs=*/
  Product : Product
  Subtract : Sum  Inputs=+-
  Subtract1 : Sum  Inputs=+-
  ln(1+activity) : Subsystem
  ln(1+rateFactor) : Subsystem
  MSR : Outport
  wires:
  Constant/1 -> Subtract/1
  rate Factor/1 -> Subtract/2
  URL/1 -> Subtract1/1
  LRL/1 -> Add2/2, Subtract1/2
  ln(1+activity)/1(Out1) -> Divide/1
  ln(1+rateFactor)/1(Out1) -> Divide/2
  Divide/1 -> Product/1
  Subtract1/1 -> Product/2
  Add2/1 -> MSR/1
  Product/1 -> Add2/1
  Subtract/1 -> ln(1+rateFactor)/1(In1)
  Activity/1 -> ln(1+activity)/1(Activity)

== system firmware/Inputs/Rate Adaptive Subsystem/Create MSR/ln(1+activity) ==
  Activity : Inport
  Add : Sum
  Constant1 : Constant
  ln : Math  Operator=log  SaturateOnIntegerOverflow=on
  Out1 : Outport
  wires:
  Activity/1 -> Add/1
  Add/1 -> ln/1
  Constant1/1 -> Add/2
  ln/1 -> Out1/1

== system firmware/Inputs/Rate Adaptive Subsystem/Create MSR/ln(1+rateFactor) ==
  In1 : Inport
  1 : Constant
  Add : Sum
  ln : Math  Operator=log  SaturateOnIntegerOverflow=on
  Out1 : Outport
  wires:
  In1/1 -> Add/1
  Add/1 -> ln/1
  1/1 -> Add/2
  ln/1 -> Out1/1

== stateflow chart firmware/Outputs/Pacing Pin Control ==
  state PreparePaceAtrium
    entry:
    %Charging C22
    VENT_PACE_CTRL = false;
    ATR_PACE_CTRL = false;
    PACING_REF_PWM = atrialShockDutyCycle;
    PACE_CHARGE_CTRL = true;
    %Discharging C21
    PACE_GND_CTRL = true;
    Z_VENT_CTRL = false;
    Z_ATR_CTRL = false;
    ATR_GND_CTRL = true;
    %All other pins
    VENT_GND_CTRL = false;
  state Default
    entry:
    %Set all pins to 0 or false
    VENT_PACE_CTRL = false;
    ATR_PACE_CTRL = false;
    PACING_REF_PWM = 0;
    PACE_CHARGE_CTRL = false;
    PACE_GND_CTRL = false;
    Z_VENT_CTRL = false;
    Z_ATR_CTRL = false;
    ATR_GND_CTRL = false;
    VENT_GND_CTRL = false;
  state PreparePaceVentricle
    entry:
    %Charging C22
    ATR_PACE_CTRL = false;
    VENT_PACE_CTRL = false;
    PACING_REF_PWM = ventricularShockDutyCycle;
    PACE_CHARGE_CTRL = true;
    %Discharging C21
    PACE_GND_CTRL = true;
    Z_ATR_CTRL = false;
    Z_VENT_CTRL = false;
    VENT_GND_CTRL = true;
    %All other pins
    ATR_GND_CTRL = false;
  state PaceVentricle
    entry:
    %Discharging C22
    PACE_CHARGE_CTRL = false;
    PACE_GND_CTRL = true;
    ATR_PACE_CTRL = false;
    ATR_GND_CTRL = false;
    Z_ATR_CTRL = false;
    Z_VENT_CTRL = false;
    VENT_GND_CTRL = false;
    VENT_PACE_CTRL = true;
    %All other pins
    PACING_REF_PWM = 0;
  state PaceAtrium
    entry:
    %Discharging C22
    PACE_CHARGE_CTRL = false;
    PACE_GND_CTRL = true;
    VENT_PACE_CTRL = false;
    VENT_GND_CTRL = false;
    Z_VENT_CTRL = false;
    Z_ATR_CTRL = false;
    ATR_GND_CTRL = false;
    ATR_PACE_CTRL = true;
    %All other pins
    PACING_REF_PWM = 0;
    exit:
  (default) -> Default
  Default -> PreparePaceVentricle [order 2] : [preparePaceVentricle]
  Default -> PreparePaceAtrium [order 1] : [preparePaceAtrium]
  PreparePaceVentricle -> Default [order 2] : [reset == true]
  PreparePaceAtrium -> Default [order 2] : [reset == true]
  PaceVentricle -> PreparePaceVentricle [order 1] : [preparePaceVentricle]
  PreparePaceVentricle -> PaceVentricle [order 1] : [paceVentricle]
  PaceAtrium -> Default [order 2] : [reset== true]
  PaceVentricle -> Default [order 2] : [reset == true]
  PaceAtrium -> PreparePaceAtrium [order 1] : [preparePaceAtrium]
  PreparePaceAtrium -> PaceAtrium [order 1] : [paceAtrium]
  data: preparePaceAtrium input; paceAtrium input; preparePaceVentricle input; paceVentricle input; ATR_GND_CTRL output; PACE_CHARGE_CTRL output; ATR_PACE_CTRL output; PACE_GND_CTRL output; PACING_REF_PWM output; VENT_GND_CTRL output; VENT_PACE_CTRL output; Z_ATR_CTRL output; Z_VENT_CTRL output; reset input; atrialShockDutyCycle input; ventricularShockDutyCycle input

== stateflow chart firmware/Serial Communication/COM IN ==
  settings: executeAtInitialization=1
  state HANDSHAKE
    entry:
    msgID = rxdata(1);
    msgTYPE = rxdata(2);
    hs_success = true;
    send_message(1);
  state POLL_REQUEST
    entry:
    send_message(2);
  state SET_TEMP_PARAM
    entry:
    temp_mode = msg(3);
    temp_LRL = msg(4);
    temp_URL = msg(5);
    temp_ARP = typecast(msg(6:7), 'uint16');
    temp_VRP = typecast(msg(8:9), 'uint16');
    temp_APW = msg(10);
    temp_VPW = msg(11);
    temp_AAmp = typecast(msg(12:15), 'single');
    temp_VAmp = typecast(msg(16:19), 'single');
    temp_ASens = typecast(msg(20:23), 'single');
    temp_VSens = typecast(msg(24:27), 'single');
    temp_AVDelay = typecast(msg(28:29), 'uint16');
    temp_rateFactor = msg(30);
    temp_actThres = msg(31);
    temp_rxnTime = msg(32);
    temp_recTime = msg(33);
    send_message(3);
  state INITIALIZE
    % Set the inital values of parameters
    entry:
    hs_success = false;
    egram_status = 0;
    mode = 0;    temp_mode = mode;
    LRL = 60;     temp_LRL = LRL;
    URL = 120;  temp_URL = URL;
    ARP = 250;  temp_ARP = ARP;
    VRP = 320;  temp_VRP = VRP;
    APW = 1;     temp_APW = APW;
    VPW = 1;     temp_VPW = VPW;
    AAmp = 5.0;   temp_AAmp = AAmp;
    VAmp = 5.0;    temp_VAmp = VAmp;
    ASens = 4.0;   temp_ASens = ASens;
    VSens = 4.0;   temp_VSens = VSens;
    AVDelay = 150; temp_AVDelay = AVDelay;
    rateFactor = 1;  temp_rateFactor = rateFactor;
    actThres = 4;    temp_actThres = actThres;
    rxnTime = 2;     temp_rxnTime = rxnTime;
    recTime = 5;     temp_recTime = recTime;
  state MESSAGE_STORAGE
    entry:
    msg = rxdata;
    msgID = msg(1);
    msgTYPE = msg(2);
  state STANDBY
    % Waiting for COM
  state SET_PERM_PARAM
    entry:
    mode = temp_mode;
    LRL = temp_LRL;
    URL = temp_URL;
    ARP = temp_ARP;
    VRP = temp_VRP;
    APW = temp_APW;
    VPW = temp_VPW;
    AAmp = temp_AAmp;
    VAmp = temp_VAmp;
    ASens = temp_ASens;
    VSens = temp_VSens;
    AVDelay = temp_AVDelay;
    rateFactor = temp_rateFactor;
    actThres = temp_actThres;
    rxnTime = temp_rxnTime;
    recTime = temp_recTime;
    send_message(4);
  state EGRAM_TOGGLE
    entry:
    egram_status = msg(3);
  (junction 53) -> (junction 92)
  (junction 92) -> STANDBY
  POLL_REQUEST -> (junction 92)
  HANDSHAKE -> (junction 92)
  SET_PERM_PARAM -> (junction 53)
  SET_TEMP_PARAM -> (junction 53)
  (junction 113) -> HANDSHAKE [order 1] : [rxdata(3) == 72 ...
      | && rxdata(4) == 101 ...
      | && rxdata(5) == 97 ...
      | && rxdata(6) == 114 ...
      | && rxdata(7) == 116 ...
      | && rxdata(8) == 70 ...
      | && rxdata(9) == 108 ...
      | && rxdata(10) == 111 ...
      | && rxdata(11) == 119]
  MESSAGE_STORAGE -> POLL_REQUEST [order 1] : [msgTYPE == hex2dec('02')]
  (default) -> INITIALIZE
  (junction 113) -> STANDBY [order 2]
  (junction 82) -> (junction 113) [order 1] : [rxdata(2) == hex2dec('01')]
  MESSAGE_STORAGE -> SET_TEMP_PARAM [order 2] : [msgTYPE == hex2dec('03')]
  INITIALIZE -> STANDBY
  STANDBY -> (junction 82) : [status == 0]
  (junction 82) -> MESSAGE_STORAGE [order 2] : [hs_success]
  (junction 82) -> (junction 87) [order 3]
  (junction 87) -> STANDBY
  MESSAGE_STORAGE -> SET_PERM_PARAM [order 3] : [msgTYPE == hex2dec('04')]
  MESSAGE_STORAGE -> (junction 87) [order 5]
  EGRAM_TOGGLE -> (junction 87)
  MESSAGE_STORAGE -> EGRAM_TOGGLE [order 4] : [msgTYPE == hex2dec('05')]
  data: rxdata input uint8; status input uint8; mode output uint8; LRL output uint8; URL output uint8; ARP output uint16; VRP output uint16; APW output uint8; VPW output uint8; AAmp output single; VAmp output single; ASens output single; VSens output single; AVDelay output uint16; rateFactor output uint8; actThres output uint8; rxnTime output uint8; recTime output uint8; temp_mode output uint8; temp_LRL output uint8; temp_URL output uint8; temp_ARP output uint16; temp_VRP output uint16; temp_APW output uint8; temp_VPW output uint8; temp_AAmp output single; temp_VAmp output single; temp_ASens output single; temp_VSens output single; msgID output; msgTYPE output; temp_AVDelay output uint16; temp_rateFactor output uint8; temp_actThres output uint8; temp_rxnTime output uint8; temp_recTime output uint8; hs_success local; msg local; egram_status output uint8
